simulink model "w2p2"  (R2020b)
settings: Solver=VariableStepAuto  StartTime=0.0  StopTime=10.0  RelTol=1e-3
values from neighbouring files (symbols this model uses):
  be = 2    [model_parameters.m]
  bv = 1    [model_parameters.m]
  Ie = 1    [model_parameters.m]
  Iv = 5    [model_parameters.m]
  muk = 1    [model_parameters.m]
  mus = 1.5    [model_parameters.m]
  R = 1    [model_parameters.m]
settings Model: Creator=WELCOME  LastModifiedBy=WELCOME

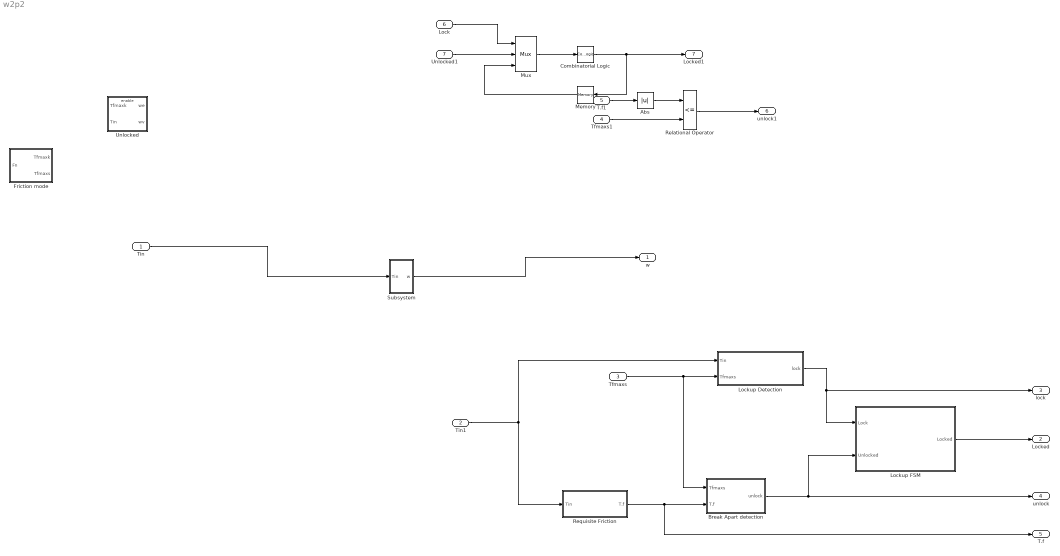
== system w2p2 ==
  Tin : Inport
  Tin1 : Inport  Port=2
  Tfmaxs : Inport  Port=3
  Tfmaxs1 : Inport  Port=4
  T.f1 : Inport  Port=5
  Lock : Inport  Port=6
  Unlocked1 : Inport  Port=7
  Abs : Abs
  Break Apart detection : Subsystem
  Combinatorial Logic : CombinatorialLogic  TruthTable=[0;1;0;0;1;1;1;0]
  Friction mode : Subsystem
  Lockup Detection : Subsystem
  Lockup FSM : Subsystem
  Memory : Memory
  Mux : Mux  Inputs=3
  Relational Operator : RelationalOperator  Operator=<=  OutDataTypeStr=boolean  RndMeth=Simplest
  Requisite Friction : Subsystem
  Subsystem : Subsystem
  Unlocked : Subsystem
  w : Outport
  Locked : Outport  Port=2
  lock : Outport  Port=3
  unlock : Outport  Port=4
  T.f : Outport  Port=5
  unlock1 : Outport  Port=6
  Locked1 : Outport  Port=7
  wires:
  Tin/1 -> Subsystem/1(Tin)
  Subsystem/1(w) -> w/1
  Requisite Friction/1(T.f) -> T.f/1, Break Apart detection/2(T.f)
  Lockup FSM/1(Locked) -> Locked/1
  Lockup Detection/1(lock) -> Lockup FSM/1(Lock), lock/1
  Break Apart detection/1(unlock) -> unlock/1, Lockup FSM/2(Unlocked)
  Tfmaxs/1 -> Break Apart detection/1(Tfmaxs), Lockup Detection/2(Tfmaxs)
  Tin1/1 -> Requisite Friction/1(Tin), Lockup Detection/1(Tin)
  T.f1/1 -> Abs/1
  Relational Operator/1 -> unlock1/1
  Abs/1 -> Relational Operator/1
  Tfmaxs1/1 -> Relational Operator/2
  Mux/1 -> Combinatorial Logic/1
  Memory/1 -> Mux/3
  Combinatorial Logic/1 -> Locked1/1, Memory/1
  Unlocked1/1 -> Mux/2
  Lock/1 -> Mux/1

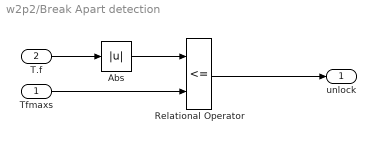
== system w2p2/Break Apart detection ==
  Tfmaxs : Inport
  T.f : Inport  Port=2
  Abs : Abs
  Relational Operator : RelationalOperator  Operator=<=  OutDataTypeStr=boolean  RndMeth=Simplest
  unlock : Outport
  wires:
  Abs/1 -> Relational Operator/1
  Tfmaxs/1 -> Relational Operator/2
  T.f/1 -> Abs/1
  Relational Operator/1 -> unlock/1

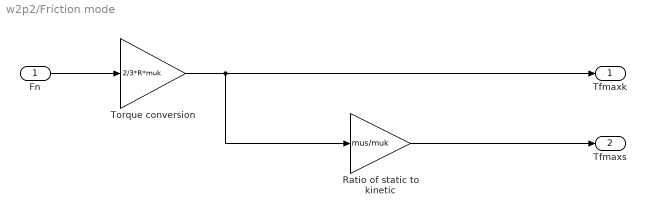
== system w2p2/Friction mode ==
  Fn : Inport
  Ratio of static to kinetic : Gain  Gain=mus/muk
  Torque conversion : Gain  Gain=2/3*R*muk
  Tfmaxk : Outport
  Tfmaxs : Outport  Port=2
  wires:
  Ratio of static to kinetic/1 -> Tfmaxs/1
  Torque conversion/1 -> Tfmaxk/1, Ratio of static to kinetic/1
  Fn/1 -> Torque conversion/1

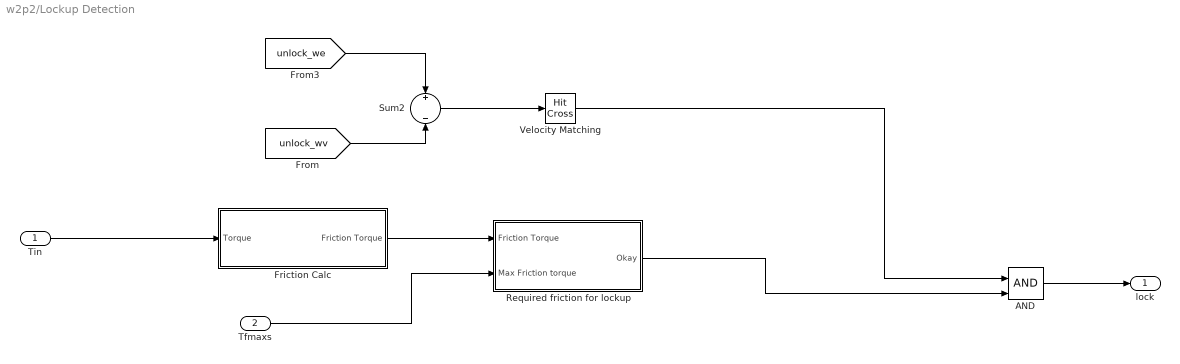
== system w2p2/Lockup Detection ==
  Tin : Inport
  Tfmaxs : Inport  Port=2
  AND : Logic  IconShape=distinctive  AllPortsSameDT=off  OutDataTypeStr=boolean
  Friction Calc : Subsystem
  Required friction for lockup : Subsystem
  Sum2 : Sum  Inputs=+|||-
  Velocity Matching : HitCross
  lock : Outport
  wires:
  AND/1 -> lock/1
  [unlock_we] -> Sum2/1
  Sum2/1 -> Velocity Matching/1
  [unlock_wv] -> Sum2/2
  Velocity Matching/1 -> AND/1
  Tfmaxs/1 -> Required friction for lockup/2(Max Friction torque)
  Tin/1 -> Friction Calc/1(Torque)
  Required friction for lockup/1(Okay) -> AND/2
  Friction Calc/1(Friction Torque) -> Required friction for lockup/1(Friction Torque)

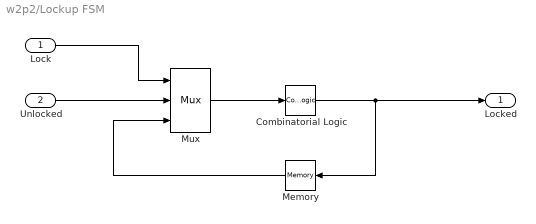
== system w2p2/Lockup FSM ==
  Lock : Inport
  Unlocked : Inport  Port=2
  Combinatorial Logic : CombinatorialLogic  TruthTable=[0;1;0;0;1;1;1;0]
  Memory : Memory
  Mux : Mux  Inputs=3
  Locked : Outport
  wires:
  Memory/1 -> Mux/3
  Mux/1 -> Combinatorial Logic/1
  Unlocked/1 -> Mux/2
  Combinatorial Logic/1 -> Locked/1, Memory/1
  Lock/1 -> Mux/1

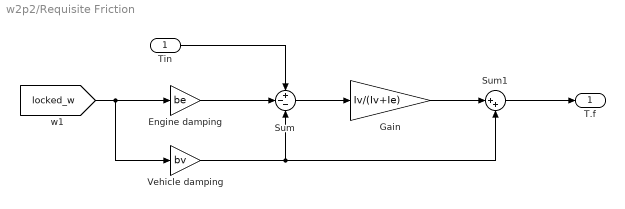
== system w2p2/Requisite Friction ==
  Tin : Inport  OutDataTypeStr=double  PortDimensions=1  SampleTime=0
  Engine damping : Gain  Gain=be
  Gain : Gain  Gain=Iv/(Iv+Ie)
  Sum : Sum  Inputs=+--
  Sum1 : Sum  Inputs=|++
  Vehicle damping : Gain  Gain=bv
  T.f : Outport  OutDataTypeStr=double  PortDimensions=1  SampleTime=0
  wires:
  Sum/1 -> Gain/1
  [locked_w] -> Engine damping/1, Vehicle damping/1
  Tin/1 -> Sum/1
  Sum1/1 -> T.f/1
  Engine damping/1 -> Sum/2
  Gain/1 -> Sum1/1
  Vehicle damping/1 -> Sum/3, Sum1/2

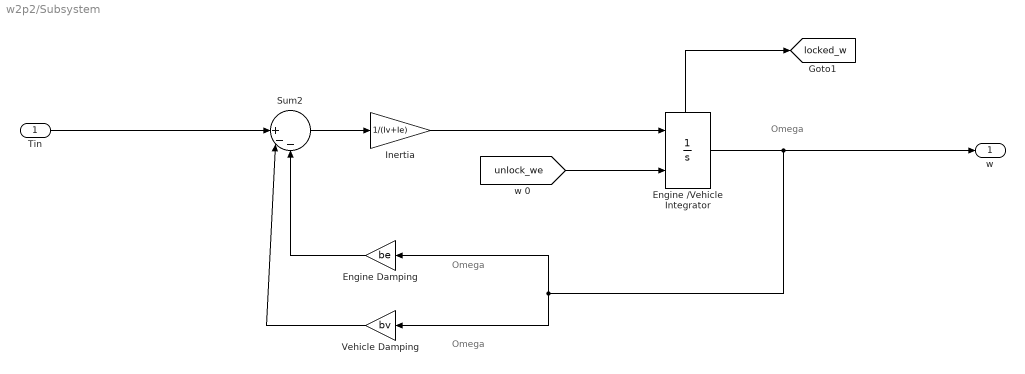
== system w2p2/Subsystem ==
  note: Omega
  note: Omega
  note: Omega
  Tin : Inport
  Engine /Vehicle Integrator : Integrator  InitialConditionSource=external  ShowStatePort=on
  Engine Damping : Gain  Gain=be
  Inertia : Gain  Gain=1/(Iv+Ie)
  Sum2 : Sum  Inputs=||+--
  Vehicle Damping : Gain  Gain=bv
  w : Outport
  tag scope: locked_w=global
  wires:
  Sum2/1 -> Inertia/1
  Inertia/1 -> Engine /Vehicle Integrator/1
  Vehicle Damping/1 -> Sum2/2
  Engine /Vehicle Integrator/1 -> w/1, Engine Damping/1, Vehicle Damping/1
  Engine Damping/1 -> Sum2/3
  Engine /Vehicle Integrator/State -> [locked_w]
  [unlock_we] -> Engine /Vehicle Integrator/2
  Tin/1 -> Sum2/1

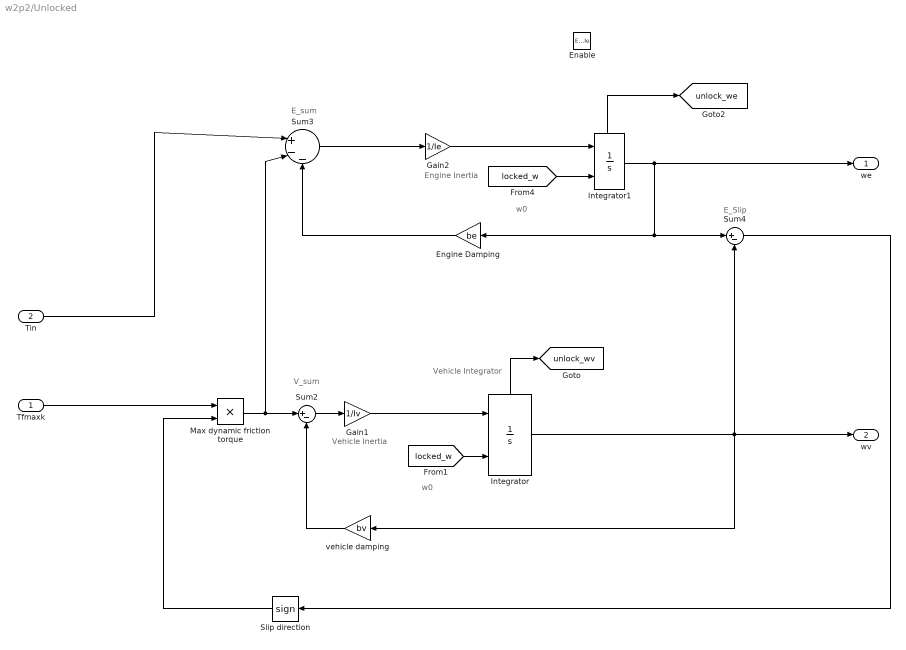
== system w2p2/Unlocked ==
  note: Vehicle Inertia
  note: V_sum
  note: Vehicle Integrator
  note: E_sum
  note: E_Slip
  note: Engine
      | Inertia
  note: w0
  note: w0
  Tfmaxk : Inport
  Tin : Inport  Port=2
  Enable : EnablePort  StatesWhenEnabling=reset
  Engine Damping : Gain  Gain=be
  Gain1 : Gain  Gain=1/Iv
  Gain2 : Gain  Gain=1/Ie
  Integrator : Integrator  InitialConditionSource=external  ShowStatePort=on
  Integrator1 : Integrator  InitialConditionSource=external  ShowStatePort=on
  Max dynamic friction torque : Product
  Slip direction : Signum
  Sum2 : Sum  Inputs=|+-
  Sum3 : Sum  Inputs=|+--
  Sum4 : Sum  Inputs=|+-
  vehicle damping : Gain  Gain=bv
  we : Outport
  wv : Outport  Port=2
  tag scope: unlock_we=global, unlock_wv=global
  wires:
  Integrator1/State -> [unlock_we]
  Tfmaxk/1 -> Max dynamic friction torque/1
  Max dynamic friction torque/1 -> Sum3/2, Sum2/1
  Integrator1/1 -> we/1, Sum4/1, Engine Damping/1
  [locked_w] -> Integrator/2
  Sum4/1 -> Slip direction/1
  Gain2/1 -> Integrator1/1
  Gain1/1 -> Integrator/1
  Integrator/State -> [unlock_wv]
  Engine Damping/1 -> Sum3/3
  vehicle damping/1 -> Sum2/2
  [locked_w] -> Integrator1/2
  Integrator/1 -> wv/1, vehicle damping/1, Sum4/2
  Sum2/1 -> Gain1/1
  Slip direction/1 -> Max dynamic friction torque/2
  Tin/1 -> Sum3/1
  Sum3/1 -> Gain2/1

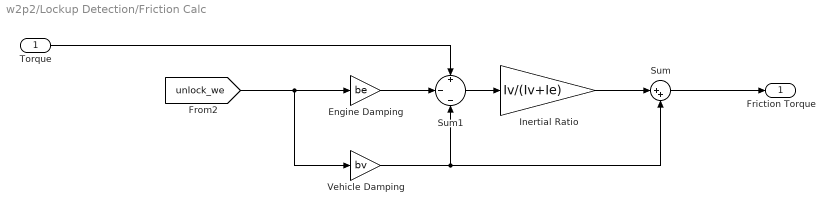
== system w2p2/Lockup Detection/Friction Calc ==
  Torque : Inport
  Engine Damping : Gain  Gain=be
  Inertial Ratio : Gain  Gain=Iv/(Iv+Ie)
  Sum : Sum  Inputs=|++
  Sum1 : Sum  Inputs=+|-|-
  Vehicle Damping : Gain  Gain=bv
  Friction Torque : Outport
  wires:
  Engine Damping/1 -> Sum1/2
  Vehicle Damping/1 -> Sum/2, Sum1/3
  [unlock_we] -> Vehicle Damping/1, Engine Damping/1
  Inertial Ratio/1 -> Sum/1
  Sum1/1 -> Inertial Ratio/1
  Torque/1 -> Sum1/1
  Sum/1 -> Friction Torque/1

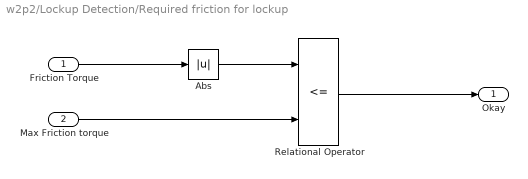
== system w2p2/Lockup Detection/Required friction for lockup ==
  Friction Torque : Inport
  Max Friction torque : Inport  Port=2
  Abs : Abs
  Relational Operator : RelationalOperator  Operator=<=  OutDataTypeStr=boolean  RndMeth=Simplest
  Okay : Outport
  wires:
  Max Friction torque/1 -> Relational Operator/2
  Friction Torque/1 -> Abs/1
  Abs/1 -> Relational Operator/1
  Relational Operator/1 -> Okay/1
